simulink model "Simulinkk"  (R2021b)
settings: Solver=ode3  StartTime=0.0  StopTime=6  FixedStep=Ts  RelTol=1e-3
PreLoadFcn:
  | %myBusDef
StartFcn:
  | % Full path to the block
  | %blk = 'Furuta_Control/Bus Creator';
  | 
  | % Attach the event listener
  | %h = add_exec_event_listener(blk, ...
  | %         'PostOutputs', @displayBusdata);
values from neighbouring files (symbols this model uses):
  alpha = J + (M + m1/3 + m2) * L1^2    (= 0.001331208)    [Constants.m]
  beta = (M + m2/3) * L2^2    (= 0.001321592)    [Constants.m]
  gamma = (M + m2/2) * L2*L1    (= 0.000684156)    [Constants.m]
  initial_state = pi    (= 3.14159265359)    [Constants.m]
  K = place(Ap,Bp,[-5 -4 -2+2j -2-2j])    [Constants.m]
  K2 = place(Ap2,Bp2,[-5 -4 -2+2j -2-2j])    [Constants.m]
  kb_m = 6.75e-4    (= 0.000675)    [Constants.m]
  kb_p = 4.7940e-04    (= 0.0004794)    [Constants.m]
  ke = 0.5    [Constants.m]
  Re = 14.5    [Constants.m]
  sigma = (M + m2/2) * g * L2    (= 0.10169046)    [Constants.m]
settings Model: Creator=Marcelo  LastModifiedBy=cadet
settings SolverCC: ZeroCrossControl=DisableAll  AlgebraicLoopSolver=TrustRegion
settings DataIOCC: ReturnWorkspaceOutputs=off
settings OptimizationCC: LifeSpan=inf
settings DebuggingCC: ParameterOverflowMsg=warning  BusObjectLabelMismatch=error  SFExecutionAtInitializationDiag=none  SFMachineParentedDataDiag=warning  ArithmeticOperatorsInVariantConditions=warning
settings HardwareCC: ProdBitPerSizeT=32  ProdBitPerPtrDiffT=32  ProdWordSize=32  ProdHWDeviceType=Specified
settings ModelReferenceCC: ModelReferenceMinAlgLoopOccurrences=on
settings SFSimCC: SimUseLocalCustomCode=off  CustomCodeUndefinedFunction=UseInterfaceOnly
settings RTWCC: RTWUseLocalCustomCode=off
settings CodeAppCC: StateflowObjectComments=on
settings ConfigComp: PLC_TargetIDE=codesys23  PLC_GenerateReport=off  PLC_LaunchReport=off

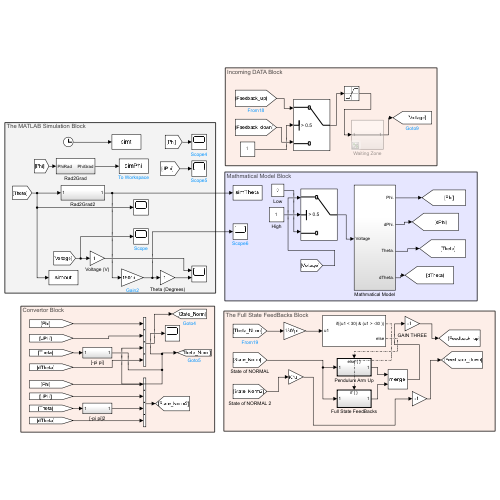
[thumbnail: Simulink's stored preview of the top-level diagram]
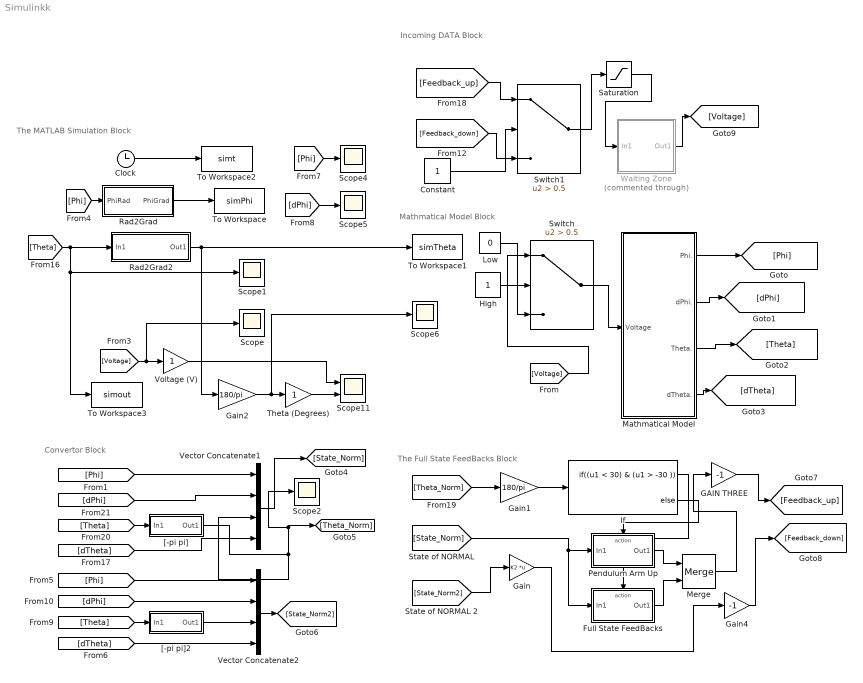
== system Simulinkk ==
  note: Convertor Block
  note: The Full State FeedBacks Block
  note: Incoming DATA Block
  note: Mathmatical Model Block
  note: The MATLAB Simulation Block
  Clock : Clock
  Constant : Constant
  Full State FeedBacks : Subsystem  TreatAsAtomicUnit=on
  GAIN THREE : Gain  Gain=-1
  Gain : Gain  Gain=K2  Multiplication=Matrix(K*u)
  Gain1 : Gain  Gain=180/pi
  Gain2 : Gain  Gain=180/pi
  Gain4 : Gain  Gain=-1
  High : Constant
  If : If  IfExpression=(u1 < 30) & (u1 > -30 )
  Low : Constant  Value=0
  "Mathmatical Model " : Subsystem
  Merge : Merge
  Pendulum Arm Up : Subsystem  TreatAsAtomicUnit=on
  Rad2Grad : Subsystem
  Rad2Grad2 : Subsystem
  Saturation : Saturate  UpperLimit=6  LowerLimit=-6
  Scope{,1..2,4..6} (6 alike) : Scope
  Scope11 : Scope  NumInputPorts=2
  Switch : Switch  Criteria=u2 > Threshold  Threshold=0.5
  Switch1 : Switch  Criteria=u2 > Threshold  Threshold=0.5
  Theta (Degrees) : Gain
  To Workspace : ToWorkspace  VariableName=simPhi  SampleTime=-1
      settings: Save2DSignal=2-D array (concatenate along first dimension)
  To Workspace1 : ToWorkspace  VariableName=simTheta  SampleTime=-1
      settings: Save2DSignal=2-D array (concatenate along first dimension)
  To Workspace2 : ToWorkspace  VariableName=simt  SampleTime=-1
      settings: Save2DSignal=2-D array (concatenate along first dimension)
  To Workspace3 : ToWorkspace  VariableName=simout  SaveFormat=Timeseries  SampleTime=-1
  Vector Concatenate1 : Concatenate  NumInputs=4
  Vector Concatenate2 : Concatenate  NumInputs=4
  Voltage (V) : Gain
  Waiting Zone : Subsystem  Commented=through
  "[-pi pi]" : Subsystem
  "[-pi pi]2" : Subsystem
  wires:
  "Mathmatical Model "/1(Phi.) -> [Phi]
  "Mathmatical Model "/2(dPhi.) -> [dPhi]
  [Voltage] -> Scope/1, Voltage (V)/1
  [Phi] -> Scope4/1
  [dPhi] -> Scope5/1
  [Theta] -> "[-pi pi]"/1(In1)
  Rad2Grad2/1(Out1) -> Gain2/1, To Workspace1/1
  Clock/1 -> To Workspace2/1
  Rad2Grad/1(PhiGrad) -> To Workspace/1
  If/2 -> Pendulum Arm Up/Action
  Pendulum Arm Up/1(Out1) -> Merge/1
  If/1 -> Full State FeedBacks/Action
  Gain2/1 -> Scope6/1, Theta (Degrees)/1
  "Mathmatical Model "/4(dTheta.) -> [dTheta]
  [dTheta] -> Vector Concatenate1/4
  Full State FeedBacks/1(Out1) -> Merge/2
  [Voltage] -> Switch/1
  High/1 -> Switch/2
  Low/1 -> Switch/3
  [Phi] -> Rad2Grad/1(PhiRad)
  Voltage (V)/1 -> Scope11/1
  "Mathmatical Model "/3(Theta.) -> [Theta]
  [dPhi] -> Vector Concatenate1/2
  [Phi] -> Vector Concatenate1/1
  Vector Concatenate1/1 -> [State_Norm]
  "[-pi pi]"/1(Out1) -> [Theta_Norm], Scope2/1, Vector Concatenate1/3
  [State_Norm] -> Full State FeedBacks/1(In1), Pendulum Arm Up/1(In1)
  [Theta_Norm] -> Gain1/1
  Gain1/1 -> If/1
  "[-pi pi]2"/1(Out1) -> Vector Concatenate2/3
  [dPhi] -> Vector Concatenate2/2
  [dTheta] -> Vector Concatenate2/4
  [Phi] -> Vector Concatenate2/1
  [Theta] -> "[-pi pi]2"/1(In1)
  Vector Concatenate2/1 -> [State_Norm2]
  [State_Norm2] -> Gain/1
  Waiting Zone/1(Out1) -> [Voltage]
  Switch1/1 -> Saturation/1
  Saturation/1 -> Waiting Zone/1(In1)
  [Feedback_up] -> Switch1/1
  [Feedback_down] -> Switch1/3
  Merge/1 -> GAIN THREE/1
  GAIN THREE/1 -> [Feedback_up]
  Constant/1 -> Switch1/2
  Switch/1 -> "Mathmatical Model "/1("Voltage ")
  Theta (Degrees)/1 -> Scope11/2
  [Theta] -> Rad2Grad2/1(In1), Scope1/1, To Workspace3/1
  Gain/1 -> Gain4/1
  Gain4/1 -> [Feedback_down]

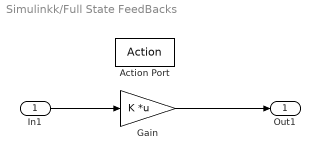
== system Simulinkk/Full State FeedBacks ==
  In1 : Inport
  Action Port : ActionPort  ActionPortLabel=if((u1 < 30) & (u1 > -30 ))
  Gain : Gain  Gain=K  Multiplication=Matrix(K*u)  ParamDataTypeStr=double  OutDataTypeStr=double
  Out1 : Outport
  wires:
  In1/1 -> Gain/1
  Gain/1 -> Out1/1

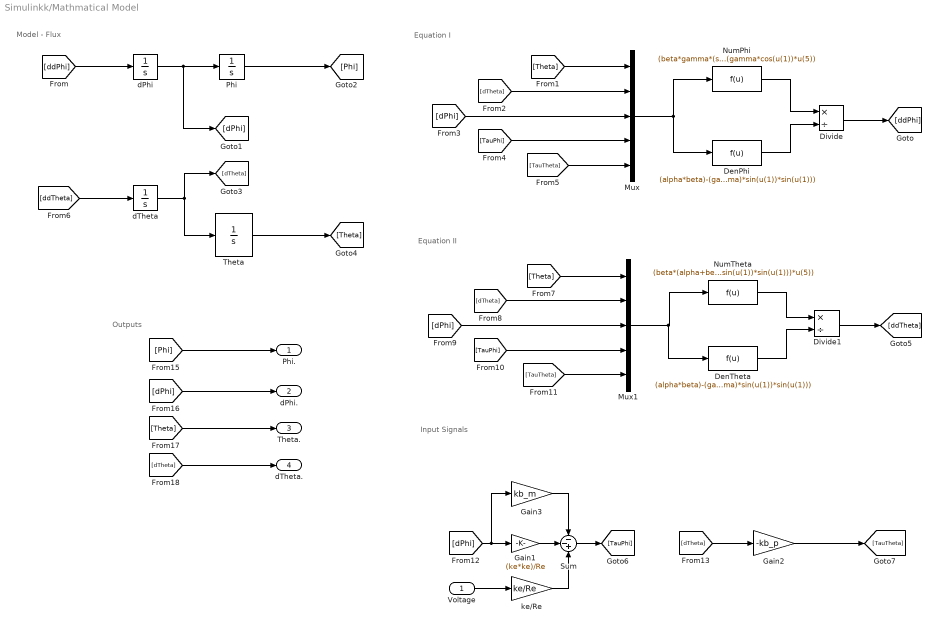
== system Simulinkk/Mathmatical Model  ==
  note: Outputs
  note: Input Signals
  note: Equation II
  note: Equation I
  note: Model - Flux
  "Voltage " : Inport
  DenPhi : Fcn  Expr=(alpha*beta)-(gamma*gamma)+((beta*beta+gamma*gamma)*sin(u(1))*sin(u(1)))
  DenTheta : Fcn  Expr=(alpha*beta)-(gamma*gamma)+((beta*beta+gamma*gamma)*sin(u(1))*sin(u(1)))
  Divide : Product  Inputs=*/
  Divide1 : Product  Inputs=*/
  Gain1 : Gain  Gain=(ke*ke)/Re
  Gain2 : Gain  Gain=-kb_p
  Gain3 : Gain  Gain=kb_m
  Mux : Mux  Inputs=5
  Mux1 : Mux  Inputs=5
  NumPhi : Fcn  Expr=(beta*gamma*(sin(u(1))*sin(u(1))-1)*sin(u(1))*u(3)*u(3))-(2*beta*beta*cos(u(1))*sin(u(1))*u(3)*u(2))+(beta*gamma*sin(u(1))*u(2)*u(2))-(gamma*sigma*cos(u(1))*sin(u(1)))+(beta*u(4))-(gamma*cos(u(1))*u(5))
  NumTheta : Fcn  Expr=(beta*(alpha+beta*sin(u(1))*sin(u(1)))*cos(u(1))*sin(u(1))*u(3)*u(3))+(2*beta*gamma*(1-sin(u(1))*sin(u(1)))*sin(u(1))*u(3)*u(2))-(gamma*gamma*cos(u(1))*sin(u(1))*u(2)*u(2))+(sigma*(alpha+beta*sin(u(1))*sin(u(1)))*sin(u(1)))-(gamma*cos(u(1))*u(4))+((alpha+beta*sin(u(1))*sin(u(1)))*u(5))
  Phi : Integrator
  Sum : Sum  Inputs=--+
  Theta : Integrator  InitialCondition=initial_state
  dPhi : Integrator
  dTheta : Integrator
  "ke/Re " : Gain  Gain=ke/Re
  Phi. : Outport
  dPhi. : Outport  Port=2
  Theta. : Outport  Port=3
  dTheta. : Outport  Port=4
  wires:
  Divide/1 -> [ddPhi]
  "ke/Re "/1 -> Sum/3
  Sum/1 -> [TauPhi]
  Gain1/1 -> Sum/2
  "Voltage "/1 -> "ke/Re "/1
  [dTheta] -> Gain2/1
  Gain3/1 -> Sum/1
  dTheta/1 -> [dTheta], Theta/1
  Theta/1 -> [Theta]
  [Theta] -> Mux1/1
  Mux1/1 -> DenTheta/1, NumTheta/1
  [dTheta] -> Mux1/2
  [dPhi] -> Mux1/3
  [TauTheta] -> Mux1/5
  [TauPhi] -> Mux1/4
  [Theta] -> Mux/1
  [TauTheta] -> Mux/5
  [TauPhi] -> Mux/4
  Phi/1 -> [Phi]
  [dPhi] -> Mux/3
  DenPhi/1 -> Divide/2
  [ddPhi] -> dPhi/1
  [ddTheta] -> dTheta/1
  dPhi/1 -> [dPhi], Phi/1
  NumTheta/1 -> Divide1/1
  NumPhi/1 -> Divide/1
  DenTheta/1 -> Divide1/2
  Mux/1 -> DenPhi/1, NumPhi/1
  [dPhi] -> Gain3/1, Gain1/1
  [dTheta] -> Mux/2
  Divide1/1 -> [ddTheta]
  [Phi] -> Phi./1
  [dPhi] -> dPhi./1
  [Theta] -> Theta./1
  [dTheta] -> dTheta./1
  Gain2/1 -> [TauTheta]

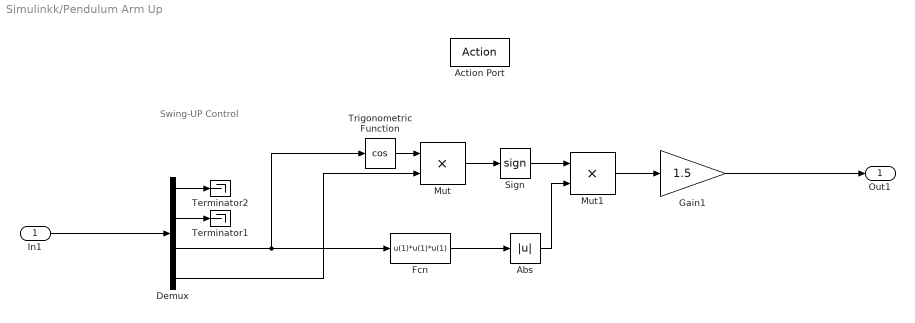
== system Simulinkk/Pendulum Arm Up ==
  note: Swing-UP Control
  In1 : Inport
  Action Port : ActionPort  ActionPortLabel=else
  Abs : Abs
  Demux : Demux
  Fcn : Fcn  Expr=u(1)*u(1)*u(1)
  Gain1 : Gain  Gain=1.5
  Mut : Product  Inputs=**
  Mut1 : Product  Inputs=**
  Sign : Signum
  Terminator1 : Terminator
  Terminator2 : Terminator
  Trigonometric Function : Trigonometry  Operator=cos
  Out1 : Outport  InitialOutput=0
  wires:
  Gain1/1 -> Out1/1
  Demux/2 -> Terminator1/1
  Demux/1 -> Terminator2/1
  Mut1/1 -> Gain1/1
  Fcn/1 -> Abs/1
  Trigonometric Function/1 -> Mut/1
  Demux/4 -> Mut/2
  Abs/1 -> Mut1/2
  Sign/1 -> Mut1/1
  Mut/1 -> Sign/1
  Demux/3 -> Fcn/1, Trigonometric Function/1
  In1/1 -> Demux/1

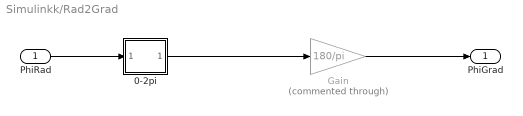
== system Simulinkk/Rad2Grad ==
  PhiRad : Inport
  0-2pi : Subsystem
  Gain : Gain  Commented=through  Gain=180/pi
  PhiGrad : Outport
  wires:
  0-2pi/1(Out1) -> Gain/1
  Gain/1 -> PhiGrad/1
  PhiRad/1 -> 0-2pi/1(In1)

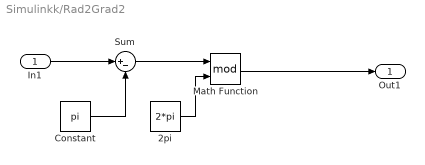
== system Simulinkk/Rad2Grad2 ==
  In1 : Inport
  2pi : Constant  Value=2*pi
  Constant : Constant  Value=pi
  Math Function : Math  Operator=mod  SignedPower=on  SaturateOnIntegerOverflow=on
  Sum : Sum  Inputs=|+-
  Out1 : Outport
  wires:
  Constant/1 -> Sum/2
  Sum/1 -> Math Function/1
  2pi/1 -> Math Function/2
  In1/1 -> Sum/1
  Math Function/1 -> Out1/1

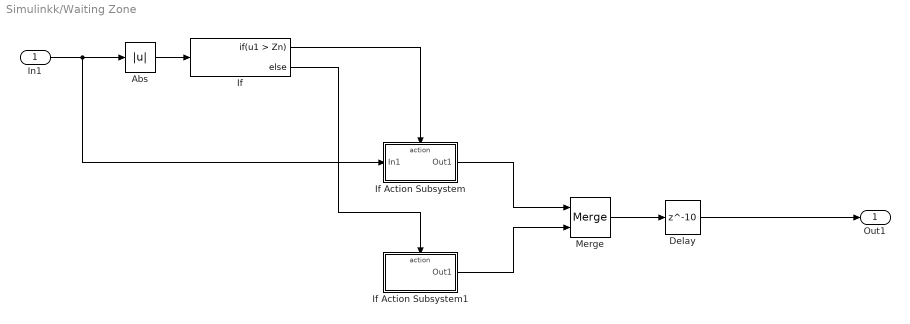
== system Simulinkk/Waiting Zone ==
  In1 : Inport
  Abs : Abs
  Delay : Delay  DelayLength=10
  If : If  IfExpression=u1 > Zn
  If Action Subsystem : Subsystem  TreatAsAtomicUnit=on
  If Action Subsystem1 : Subsystem  TreatAsAtomicUnit=on
  Merge : Merge
  Out1 : Outport
  wires:
  Delay/1 -> Out1/1
  Merge/1 -> Delay/1
  If Action Subsystem1/1(Out1) -> Merge/2
  If Action Subsystem/1(Out1) -> Merge/1
  If/2 -> If Action Subsystem1/Action
  If/1 -> If Action Subsystem/Action
  Abs/1 -> If/1
  In1/1 -> Abs/1, If Action Subsystem/1(In1)

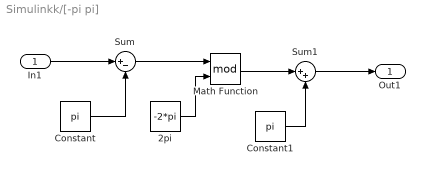
== system Simulinkk/[-pi pi] ==
  In1 : Inport
  2pi : Constant  Value=-2*pi
  Constant : Constant  Value=pi
  Constant1 : Constant  Value=pi
  Math Function : Math  Operator=mod  SignedPower=on  SaturateOnIntegerOverflow=on
  Sum : Sum  Inputs=|+-
  Sum1 : Sum  Inputs=|++
  Out1 : Outport
  wires:
  2pi/1 -> Math Function/2
  In1/1 -> Sum/1
  Sum/1 -> Math Function/1
  Constant/1 -> Sum/2
  Constant1/1 -> Sum1/2
  Sum1/1 -> Out1/1
  Math Function/1 -> Sum1/1

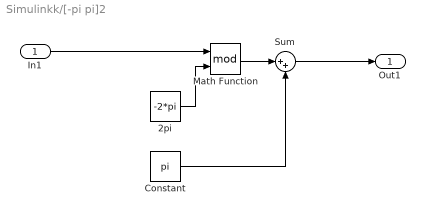
== system Simulinkk/[-pi pi]2 ==
  In1 : Inport
  2pi : Constant  Value=-2*pi
  Constant : Constant  Value=pi
  Math Function : Math  Operator=mod  SignedPower=on  SaturateOnIntegerOverflow=on
  Sum : Sum  Inputs=|++
  Out1 : Outport
  wires:
  2pi/1 -> Math Function/2
  In1/1 -> Math Function/1
  Math Function/1 -> Sum/1
  Constant/1 -> Sum/2
  Sum/1 -> Out1/1

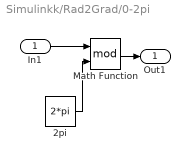
== system Simulinkk/Rad2Grad/0-2pi ==
  In1 : Inport
  2pi : Constant  Value=2*pi
  Math Function : Math  Operator=mod  SignedPower=on  SaturateOnIntegerOverflow=on
  Out1 : Outport
  wires:
  2pi/1 -> Math Function/2
  Math Function/1 -> Out1/1
  In1/1 -> Math Function/1

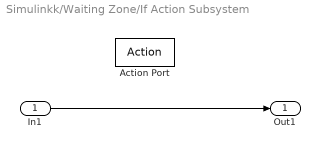
== system Simulinkk/Waiting Zone/If Action Subsystem ==
  In1 : Inport
  Action Port : ActionPort  ActionPortLabel=if { }
  Out1 : Outport
  wires:
  In1/1 -> Out1/1

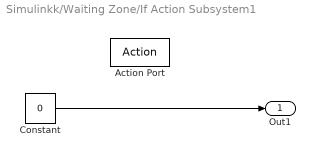
== system Simulinkk/Waiting Zone/If Action Subsystem1 ==
  Action Port : ActionPort  ActionPortLabel=else { }
  Constant : Constant  Value=0
  Out1 : Outport
  wires:
  Constant/1 -> Out1/1
